simulink model "N3Z_tonetest14b"  (R2014b)
settings: Solver=ode3  SolverMode=SingleTasking  StartTime=0.0  StopTime=1e-4  FixedStep=fpgaclk  RelTol=1e-3
PreLoadFcn:
  | %fpgaclk=1/32.768e6
  | fpgaclk=1/49.162e6
  | 
  | SerialData=[1,zeros(1,11),1,0,0,1]
  | load ../N3workingG/window
  | win=win';  %Go back to using flatter and wider windowed sync function
  | %load ../N3workingG/hanning    %use Hahn window
  | 
  | load ../N3workingG/PREemphasis   %For pre-empasis and deemphasis FIRs
  | 
  | %LUT3=xls2LUT2('../IQI_Qdemod.xls'); LUT3
  | load ../N3workingG/LUT3
  | load ../N3workingG/FIRiq2
  | % xls2LUT
  | 
  | GetProgFiles
  | 
  | PinAssignments    %Get Pin references for TE0722
  | 
  | 
  | 
  | 
  | 
  | %LCD
  | LCDdata=[LCD_D7,LCD_D6,LCD_D5,LCD_D4,LCD_D3,LCD_D2,LCD_D1,LCD_D0] %Note MSB...LSB!
  | LCDctrl=[LCD_E,LCD_RW,LCD_RS];
  | 
  | %for RS232 on pins 3 and 5 of USBB
  | 
  | %BT chip connections for WT12
  | 
  | RX_BT=RXD
  | TX_BT=TXD
  | 
  | RST_BB=RES
  | 
  | %PCMC=PCMC
  | %PCMS=PCMS
  | %PCMI=PCMI
  | %PCMO=PCMO
  | 
  | %Aliases:
  | SRDBT=PCMI
  | STDBT=PCMO
  | SCLK_BT=PCMC
  | SFS_BT=PCMS
  | 
  | %ADC control
  | 
  | %SDOA=SDOA
  | %SDOB=SDOB
  | %SCK=SCK
  | CONV=Csbar
  | CAL=Cal
  | 
  | ADC_G=[ADC_G3,ADC_G2,ADC_G1,ADC_G0]
  | %PD settings hard coded now
  | 
  | %%%%%%
  | TX_LOW=TX_Low
  | ... (+11 lines)
StartFcn:
  | SerialData=[1,zeros(1,11),1,0,0,1]
values from neighbouring files (symbols this model uses):
  ADC_G0 = {'P10'}    [PinAssignments.m]
  ADC_G1 = {'P11'}    [PinAssignments.m]
  ADC_G2 = {'N14'}    [PinAssignments.m]
  ADC_G3 = {'M11'}    [PinAssignments.m]
  Cal = {'L12'}    [PinAssignments.m]
  Csbar = {'M12'}    [PinAssignments.m]
  LCD_D0 = {'J13'}    [PinAssignments.m]
  LCD_D1 = {'J14'}    [PinAssignments.m]
  LCD_D2 = {'F15'}    [PinAssignments.m]
  LCD_D3 = {'H14'}    [PinAssignments.m]
  LCD_D4 = {'G12'}    [PinAssignments.m]
  LCD_D5 = {'L15'}    [PinAssignments.m]
  LCD_D6 = {'M14'}    [PinAssignments.m]
  LCD_D7 = {'K15'}    [PinAssignments.m]
  PCMC = {'H11'}    [PinAssignments.m]
  PCMI = {'H12'}    [PinAssignments.m]
  PCMO = {'N13'}    [PinAssignments.m]
  PCMS = {'M10'}    [PinAssignments.m]
  RES = {'G11'}    [PinAssignments.m]
  RXD = {'H13'}    [PinAssignments.m]
  TX_Low = {'P15'}    [PinAssignments.m]
  TXD = {'P13'}    [PinAssignments.m]
undefined symbols (not defined in the file or in its folder): AXI4, FIRRX, FIRTX, Lite
libraries: xbsIndex_r4 x1214, MyFunctions x43
(part 5 of 9)

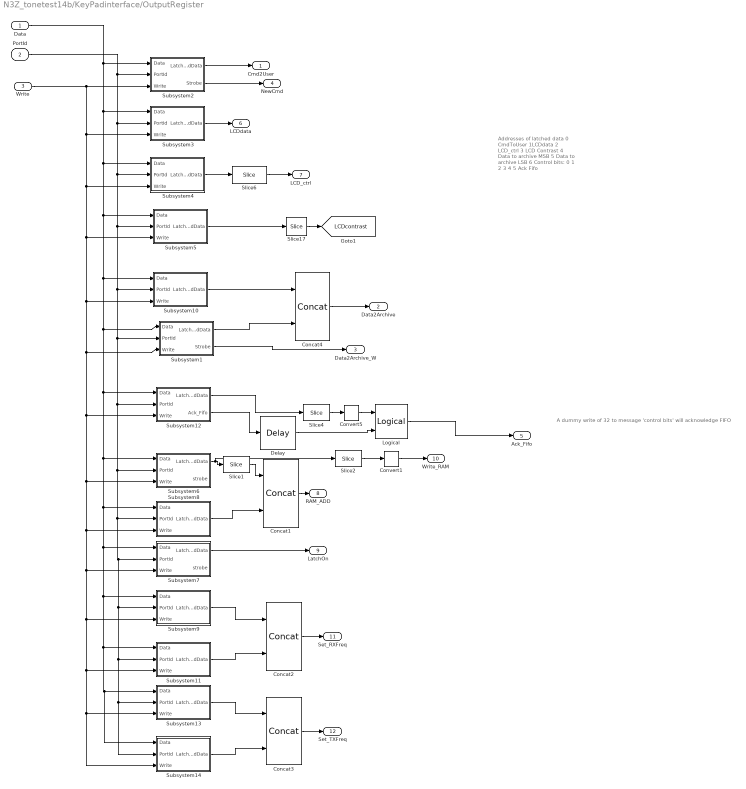
== system N3Z_tonetest14b/KeyPadinterface/OutputRegister ==
  note: A dummy write of 32 to message 'control bits' will acknowledge FIFO
  note: Addresses of latched data
      | 0 CmdToUser
      | 1LCDdata
      | 2 LCD_ctrl
      | 3 LCD Contrast
      | 4 Data to archive MSB
      | 5 Data to archive LSB
      | 6 Control bits:
      | 	0
      | 	1
      | 	2
      | 	3
      | 	4
      | 	5 Ack Fifo
  Data : Inport
  PortId : Inport  Port=2
  Write : Inport  Port=3
  Concat{1..4} (4 alike) : xbsIndex_r4/Concat  num_inputs=2  dbl_ovrd=off  block_type=concat
      settings: block_version=8.2.02
  Convert1 : xbsIndex_r4/Convert  gui_display_data_type=Fixed-point  arith_type=Boolean  n_bits=16  bin_pt=0  float_type=Single  exp_bits=8  fraction_bits=24  quantization=Truncate  overflow=Wrap  en=off  latency=0  pipeline=off  dbl_ovrd=off  block_type=convert
      settings: xl_area=[0, 0, 0, 0, 0, 0, 0]  block_version=VER_STRING_GOES_HERE
  Convert5 : xbsIndex_r4/Convert  gui_display_data_type=Fixed-point  arith_type=Boolean  n_bits=16  bin_pt=0  float_type=Single  exp_bits=8  fraction_bits=24  quantization=Truncate  overflow=Wrap  en=off  latency=0  pipeline=off  dbl_ovrd=off  block_type=convert
      settings: xl_area=[0, 0, 0, 0, 0, 0, 0]  block_version=VER_STRING_GOES_HERE
  Delay : xbsIndex_r4/Delay  rst=off  infoeditControl=Selection of Reset will increase slice count due to use of real FFs and instead of SRLs  en=off  latency=1  reg_retiming=off  dbl_ovrd=off  block_type=delay
      settings: infoedit=Hardware notes: A delay line is a chain, each link of which is an SRL16 followed by a flip-flop. If register retiming is enabled, the delay line is a chain of flip-flops.  block_version=8.2.02
  Logical : xbsIndex_r4/Logical  logical_function=AND  inputs=2  en=off  latency=0  precision=Full  arith_type=Unsigned  n_bits=16  bin_pt=0  align_bp=on  dbl_ovrd=off  block_type=logical
      settings: block_version=8.2.02
  Slice1 : xbsIndex_r4/Slice  nbits=2  boolean_output=off  mode=Lower Bit Location + Width  bit1=-16  base1=MSB of Input  bit0=0  base0=LSB of Input  dbl_ovrd=off  block_type=slice
      settings: block_version=VER_STRING_GOES_HERE
  Slice17 : xbsIndex_r4/Slice  nbits=6  boolean_output=off  mode=Lower Bit Location + Width  bit1=3  base1=MSB of Input  bit0=0  base0=LSB of Input  dbl_ovrd=off  block_type=slice
      settings: block_version=8.2.02
  Slice2 : xbsIndex_r4/Slice  nbits=1  boolean_output=off  mode=Lower Bit Location + Width  bit1=-16  base1=MSB of Input  bit0=2  base0=LSB of Input  dbl_ovrd=off  block_type=slice
      settings: block_version=VER_STRING_GOES_HERE
  Slice4 : xbsIndex_r4/Slice  nbits=1  boolean_output=off  mode=Lower Bit Location + Width  bit1=-16  base1=MSB of Input  bit0=5  base0=LSB of Input  dbl_ovrd=off  block_type=slice
      settings: block_version=VER_STRING_GOES_HERE
  Slice6 : xbsIndex_r4/Slice  nbits=4  boolean_output=off  mode=Lower Bit Location + Width  bit1=3  base1=MSB of Input  bit0=0  base0=LSB of Input  dbl_ovrd=off  block_type=slice
      settings: block_version=8.2.02
  Subsystem1 : Subsystem
  Subsystem10 : Subsystem
  Subsystem11 : Subsystem
  Subsystem12 : Subsystem
  Subsystem13 : Subsystem
  Subsystem14 : Subsystem
  Subsystem2 : Subsystem
  Subsystem3 : Subsystem
  Subsystem4 : Subsystem
  Subsystem5 : Subsystem
  Subsystem6 : Subsystem
  Subsystem7 : Subsystem
  Subsystem8 : Subsystem
  Subsystem9 : Subsystem
  Cmd2User : Outport
  Data2Archive : Outport  Port=2
  Data2Archive_W : Outport  Port=3
  NewCmd : Outport  Port=4
  Ack_Fifo : Outport  Port=5
  LCDdata : Outport  Port=6
  LCD_ctrl : Outport  Port=7
  RAM_ADD : Outport  Port=8
  LatchOn : Outport  Port=9
  Write_RAM : Outport  Port=10
  Set_RXFreq : Outport  Port=11
  Set_TXFreq : Outport  Port=12
  tag scope: LCDcontrast=global
  wires:
  PortId/1 -> Subsystem2/2(PortId), Subsystem3/2(PortId), Subsystem4/2(PortId), Subsystem5/2(PortId), Subsystem10/2(PortId), Subsystem1/2(PortId), Subsystem12/2(PortId), Subsystem8/2(PortId), Subsystem9/2(PortId), Subsystem11/2(PortId), Subsystem13/2(PortId), Subsystem14/2(PortId), Subsystem7/2(PortId), Subsystem6/2(PortId)
  Data/1 -> Subsystem2/1(Data), Subsystem3/1(Data), Subsystem4/1(Data), Subsystem5/1(Data), Subsystem10/1(Data), Subsystem1/1(Data), Subsystem12/1(Data), Subsystem8/1(Data), Subsystem14/1(Data), Subsystem13/1(Data), Subsystem11/1(Data), Subsystem9/1(Data), Subsystem7/1(Data), Subsystem6/1(Data)
  Write/1 -> Subsystem2/3(Write), Subsystem3/3(Write), Subsystem4/3(Write), Subsystem5/3(Write), Subsystem10/3(Write), Subsystem1/3(Write), Subsystem12/3(Write), Subsystem6/3(Write), Subsystem8/3(Write), Subsystem9/3(Write), Subsystem11/3(Write), Subsystem13/3(Write), Subsystem14/3(Write), Subsystem7/3(Write)
  Subsystem2/1(LatchedData) -> Cmd2User/1
  Concat4/1 -> Data2Archive/1
  Subsystem10/1(LatchedData) -> Concat4/1
  Subsystem12/1(LatchedData) -> Slice4/1
  Slice4/1 -> Convert5/1
  Convert5/1 -> Logical/1
  Subsystem2/2(Strobe) -> NewCmd/1
  Subsystem12/2(Ack_Fifo) -> Delay/1
  Logical/1 -> Ack_Fifo/1
  Delay/1 -> Logical/2
  Subsystem3/1(LatchedData) -> LCDdata/1
  Subsystem4/1(LatchedData) -> Slice6/1
  Slice6/1 -> LCD_ctrl/1
  Subsystem5/1(LatchedData) -> Slice17/1
  Slice17/1 -> [LCDcontrast]
  Subsystem1/2(Strobe) -> Data2Archive_W/1
  Subsystem1/1(LatchedData) -> Concat4/2
  Subsystem7/1(LatchedData) -> LatchOn/1
  Subsystem6/1(LatchedData) -> Slice1/1, Slice2/1
  Slice1/1 -> Concat1/1
  Subsystem8/1(LatchedData) -> Concat1/2
  Concat1/1 -> RAM_ADD/1
  Slice2/1 -> Convert1/1
  Convert1/1 -> Write_RAM/1
  Subsystem9/1(LatchedData) -> Concat2/1
  Subsystem11/1(LatchedData) -> Concat2/2
  Concat2/1 -> Set_RXFreq/1
  Subsystem13/1(LatchedData) -> Concat3/1
  Subsystem14/1(LatchedData) -> Concat3/2
  Concat3/1 -> Set_TXFreq/1

== system N3Z_tonetest14b/LoranPulsedetect/FastLevelMonitor ==
  note: Add 13 bits above and below to get ~2.5s time constant
  note: Feb 2011 added 1 bit to AddSub unit
  note: Increase Threshold 25%
  In1 : Inport
  En : Inport  Port=2
  AddSub : xbsIndex_r4/AddSub  mode=Addition or Subtraction  use_carryin=off  use_carryout=off  en=off  latency=0  precision=User Defined  arith_type=Unsigned  n_bits=13  bin_pt=0  quantization=Truncate  overflow=Wrap  use_behavioral_HDL=off  hw_selection=Fabric  pipelined=off  dbl_ovrd=off  block_type=addsub
      settings: block_version=12.2
  AddSub1 : xbsIndex_r4/AddSub  mode=Addition  use_carryin=off  use_carryout=off  en=off  latency=0  precision=User Defined  arith_type=Unsigned  n_bits=8  bin_pt=0  quantization=Truncate  overflow=Wrap  use_behavioral_HDL=off  hw_selection=Fabric  pipelined=off  dbl_ovrd=off  block_type=addsub
      settings: block_version=12.2
  Convert : xbsIndex_r4/Convert  gui_display_data_type=Fixed-point  arith_type=Boolean  n_bits=16  bin_pt=14  float_type=Single  exp_bits=8  fraction_bits=24  quantization=Truncate  overflow=Wrap  en=off  latency=0  pipeline=off  dbl_ovrd=off  block_type=convert
      settings: block_version=12.2
  Convert1 : xbsIndex_r4/Convert  gui_display_data_type=Fixed-point  arith_type=Boolean  n_bits=16  bin_pt=14  float_type=Single  exp_bits=8  fraction_bits=24  quantization=Truncate  overflow=Wrap  en=off  latency=0  pipeline=off  dbl_ovrd=off  block_type=convert
      settings: block_version=12.2
  Convert2 : xbsIndex_r4/Convert  gui_display_data_type=Fixed-point  arith_type="Signed  (2's comp)"  n_bits=8  bin_pt=0  float_type=Single  exp_bits=8  fraction_bits=24  quantization=Truncate  overflow=Wrap  en=off  latency=0  pipeline=off  dbl_ovrd=off  block_type=convert
      settings: block_version=12.2
  Counter : xbsIndex_r4/Counter  cnt_type=Free Running  cnt_to=Inf  operation=Up  start_count=0  cnt_by_val=1  arith_type=Unsigned  n_bits=8  bin_pt=0  load_pin=off  rst=off  en=on  explicit_period=on  period=fpgaclk  use_behavioral_HDL=off  implementation=Fabric  dbl_ovrd=off  block_type=counter
      settings: block_version=12.2
  Monostable : MyFunctions/Monostable
  Register : xbsIndex_r4/Register  init=0  rst=on  en=on  dbl_ovrd=off  block_type=register
      settings: block_version=12.2
  Register1 : xbsIndex_r4/Register  init=0  rst=off  en=on  dbl_ovrd=off  block_type=register
      settings: block_version=12.2
  Slice1 : xbsIndex_r4/Slice  nbits=1  boolean_output=off  mode=Upper Bit Location + Width  bit1=0  base1=MSB of Input  bit0=0  base0=LSB of Input  dbl_ovrd=off  block_type=slice
      settings: block_version=12.2
  Slice2 : xbsIndex_r4/Slice  nbits=1  boolean_output=off  mode=Upper Bit Location + Width  bit1=0  base1=MSB of Input  bit0=0  base0=LSB of Input  dbl_ovrd=off  block_type=slice
      settings: block_version=12.2
  Slice3 : xbsIndex_r4/Slice  nbits=8  boolean_output=off  mode=Upper Bit Location + Width  bit1=0  base1=MSB of Input  bit0=0  base0=LSB of Input  dbl_ovrd=off  block_type=slice
      settings: block_version=12.2
  Slice4 : xbsIndex_r4/Slice  nbits=8  boolean_output=off  mode=Upper Bit Location + Width  bit1=-1  base1=MSB of Input  bit0=0  base0=LSB of Input  dbl_ovrd=off  block_type=slice
      settings: block_version=12.2
  Slice5 : xbsIndex_r4/Slice  nbits=6  boolean_output=off  mode=Upper Bit Location + Width  bit1=0  base1=MSB of Input  bit0=0  base0=LSB of Input  dbl_ovrd=off  block_type=slice
      settings: block_version=12.2
  SignalLevel : Outport
  wires:
  In1/1 -> Slice1/1, Slice4/1
  AddSub/1 -> Register/1
  En/1 -> Register/3, Counter/1
  Slice1/1 -> Convert/1
  Convert/1 -> AddSub/3
  Register/1 -> AddSub/1, Slice3/1, Slice5/1
  Counter/1 -> Slice2/1
  Monostable/1 -> Convert1/1
  Convert1/1 -> Register/2, Register1/2
  Slice2/1 -> Monostable/1
  Register1/1 -> SignalLevel/1
  Slice4/1 -> Convert2/1
  Convert2/1 -> AddSub/2
  Slice3/1 -> AddSub1/1
  Slice5/1 -> AddSub1/2
  AddSub1/1 -> Register1/1

== system N3Z_tonetest14b/LoranPulsedetect/LoranTrigger ==
  note: Divides unsigned number by 2
  LoranSignal : Inport
  Thresh : Inport  Port=2
  Relational : xbsIndex_r4/Relational  mode=a>b  op_type=Bool  en=off  latency=1  dbl_ovrd=off  block_type=relational
      settings: block_version=12.2
  Slice : xbsIndex_r4/Slice  nbits=7  boolean_output=off  mode=Upper Bit Location + Width  bit1=0  base1=MSB of Input  bit0=0  base0=LSB of Input  dbl_ovrd=off  block_type=slice
      settings: block_version=12.2
  Trig : Outport
  wires:
  Slice/1 -> Relational/2
  LoranSignal/1 -> Relational/1
  Relational/1 -> Trig/1
  Thresh/1 -> Slice/1

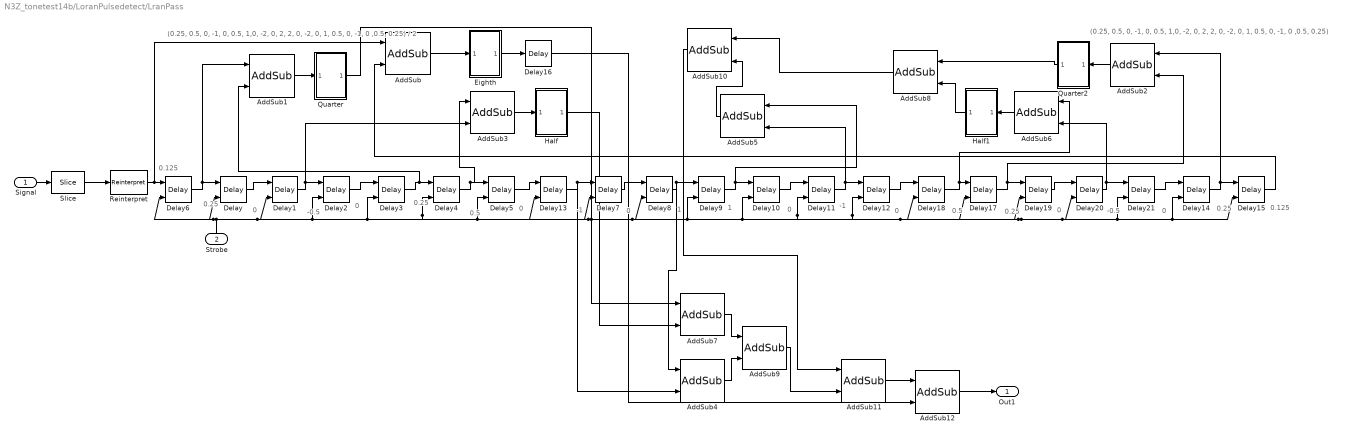
== system N3Z_tonetest14b/LoranPulsedetect/LranPass ==
  note: (0.25, 0.5, 0, -1, 0, 0.5, 1,0, -2, 0, 2, 2, 0, -2, 0, 1, 0.5, 0, -1, 0 ,0.5, 0.25) / 2
  note: (0.25, 0.5, 0, -1, 0, 0.5, 1,0, -2, 0, 2, 2, 0, -2, 0, 1, 0.5, 0, -1, 0 ,0.5, 0.25)
  note: 0.125
  note: 0.25
  note: 0
  note: -0.5
  note: 0
  note: 0.25
  note: 0.5
  note: 0
  note: -1
  note: 0
  note: 1
  note: 1
  note: 0
  note: -1
  note: 0
  note: 0.5
  note: 0.25
  note: 0
  note: -0.5
  note: 0
  note: 0.25
  note: 0.125
  Signal : Inport
  Strobe : Inport  Port=2
  AddSub{,1,7..10} (6 alike) : xbsIndex_r4/AddSub  mode=Addition  use_carryin=off  use_carryout=off  en=off  latency=1  precision=Full  arith_type=Unsigned  n_bits=16  bin_pt=14  quantization=Truncate  overflow=Wrap  use_behavioral_HDL=off  hw_selection=Fabric  pipelined=off  dbl_ovrd=off  block_type=addsub
      settings: block_version=12.2
  AddSub11 : xbsIndex_r4/AddSub  mode=Addition  use_carryin=off  use_carryout=off  en=off  latency=1  precision=User Defined  arith_type="Signed  (2's comp)"  n_bits=9  bin_pt=0  quantization=Truncate  overflow=Wrap  use_behavioral_HDL=off  hw_selection=Fabric  pipelined=off  dbl_ovrd=off  block_type=addsub
      settings: block_version=12.2
  AddSub12 : xbsIndex_r4/AddSub  mode=Addition  use_carryin=off  use_carryout=off  en=off  latency=1  precision=User Defined  arith_type="Signed  (2's comp)"  n_bits=9  bin_pt=0  quantization=Truncate  overflow=Wrap  use_behavioral_HDL=off  hw_selection=Fabric  pipelined=off  dbl_ovrd=off  block_type=addsub
      settings: block_version=12.2
  AddSub2 : xbsIndex_r4/AddSub  mode=Addition  use_carryin=off  use_carryout=off  en=off  latency=0  precision=Full  arith_type=Unsigned  n_bits=16  bin_pt=14  quantization=Truncate  overflow=Wrap  use_behavioral_HDL=off  hw_selection=Fabric  pipelined=off  dbl_ovrd=off  block_type=addsub
      settings: block_version=12.2
  AddSub{3..6} (4 alike) : xbsIndex_r4/AddSub  mode=Subtraction  use_carryin=off  use_carryout=off  en=off  latency=1  precision=Full  arith_type=Unsigned  n_bits=16  bin_pt=14  quantization=Truncate  overflow=Wrap  use_behavioral_HDL=off  hw_selection=Fabric  pipelined=off  dbl_ovrd=off  block_type=addsub
      settings: block_version=12.2
  Delay{,1..15,17..21} (21 alike) : xbsIndex_r4/Delay  rst=off  infoeditControl=Selection of Reset will increase slice count due to use of real FFs and instead of SRLs  en=on  latency=1  reg_retiming=off  dbl_ovrd=off  block_type=delay
      settings: block_version=12.2
  Delay16 : xbsIndex_r4/Delay  rst=off  infoeditControl=Selection of Reset will increase slice count due to use of real FFs and instead of SRLs  en=off  latency=3  reg_retiming=off  dbl_ovrd=off  block_type=delay
      settings: block_version=12.2
  Eighth : Subsystem
  Half : Subsystem
  Half1 : Subsystem
  Quarter : Subsystem
  Quarter2 : Subsystem
  Reinterpret : xbsIndex_r4/Reinterpret  force_arith_type=on  arith_type="Signed  (2's comp)"  force_bin_pt=off  bin_pt=0  block_type=reinterpret
      settings: infoedit="Changes signal type without altering the binary representation.   You can changed the signal between signed and unsigned, and relocate the binary point.<br><br>Hardware notes: In hardware this block costs nothing.<br><br>Example:  Suppose the input is 6 bits wide, signed, with 2 fractional bits, and the output is forced to unsigned with 0 fractional bits.  Then an input of -2.0 (1110.00 in binary 2's complement) becomes an output of 56 (111000 in binary)."  block_version=12.2
  Slice : xbsIndex_r4/Slice  nbits=8  boolean_output=off  mode=Upper Bit Location + Width  bit1=0  base1=MSB of Input  bit0=0  base0=LSB of Input  dbl_ovrd=off  block_type=slice
      settings: block_version=12.2
  Out1 : Outport
  wires:
  Delay6/1 -> Delay/1, AddSub1/1
  Delay/1 -> Delay1/1
  Delay1/1 -> Delay2/1, AddSub3/2
  Delay2/1 -> Delay3/1
  Delay3/1 -> Delay4/1, AddSub1/2
  Delay4/1 -> Delay5/1, AddSub3/1
  Strobe/1 -> Delay6/2, Delay/2, Delay1/2, Delay2/2, Delay3/2, Delay4/2, Delay5/2, Delay13/2, Delay7/2, Delay8/2, Delay9/2, Delay10/2, Delay11/2, Delay12/2, Delay18/2, Delay17/2, Delay19/2, Delay20/2, Delay21/2, Delay14/2, Delay15/2
  Signal/1 -> Slice/1
  Delay13/1 -> Delay7/1, AddSub4/2
  Delay7/1 -> Delay8/1
  Delay8/1 -> Delay9/1, AddSub4/1
  Delay9/1 -> Delay10/1, AddSub5/1
  Delay10/1 -> Delay11/1
  Delay11/1 -> Delay12/1, AddSub5/2
  Delay5/1 -> Delay13/1
  Slice/1 -> Reinterpret/1
  Delay17/1 -> Delay19/1, AddSub2/2
  Delay19/1 -> Delay20/1
  Delay20/1 -> Delay21/1, AddSub6/2
  Delay21/1 -> Delay14/1
  Delay14/1 -> Delay15/1, AddSub2/1
  Delay15/1 -> AddSub/2
  Delay18/1 -> Delay17/1, AddSub6/1
  Delay12/1 -> Delay18/1
  Reinterpret/1 -> Delay6/1, AddSub/1
  AddSub/1 -> Eighth/1(In1)
  AddSub2/1 -> Quarter2/1(In1)
  AddSub1/1 -> Quarter/1(In1)
  AddSub6/1 -> Half1/1(In1)
  AddSub3/1 -> Half/1(In1)
  Quarter/1(Out1) -> AddSub7/1
  Half/1(Out1) -> AddSub7/2
  Half1/1(Out1) -> AddSub8/2
  AddSub7/1 -> AddSub9/1
  AddSub4/1 -> AddSub9/2
  AddSub8/1 -> AddSub10/1
  AddSub5/1 -> AddSub10/2
  AddSub10/1 -> AddSub11/1
  AddSub9/1 -> AddSub11/2
  Eighth/1(Out1) -> Delay16/1
  AddSub11/1 -> AddSub12/1
  Delay16/1 -> AddSub12/2
  AddSub12/1 -> Out1/1
  Quarter2/1(Out1) -> AddSub8/1

== system N3Z_tonetest14b/SSBmodulator /RampGen ==
  note: Added 8 bits to get more precission on phase determination
  In1 : Inport
  Accumulator : xbsIndex_r4/Accumulator  operation=Add  n_bits=21  overflow=Wrap  scale=1  rst=off  hasbypass=off  infoeditControl=reset for floating point data type must be asserted for a minimum of 2 cycles  en=off  latency=0  msb_inp=100  msb=100  lsb=-100  use_behavioral_HDL=on  implementation=Fabric  dbl_ovrd=off  block_type=accum
      settings: block_version=VER_STRING_GOES_HERE
  Slice : xbsIndex_r4/Slice  nbits=17  boolean_output=off  mode=Upper Bit Location + Width  bit1=0  base1=MSB of Input  bit0=0  base0=LSB of Input  dbl_ovrd=off  block_type=slice
      settings: block_version=VER_STRING_GOES_HERE
  Out1 : Outport
  wires:
  Accumulator/1 -> Slice/1
  In1/1 -> Accumulator/1
  Slice/1 -> Out1/1

== system N3Z_tonetest14b/SSBmodulator /Subsystem ==
  note: Ramp from -2^15 to +2^15
  In1 : Inport
  In3 : Inport  Port=2
  AddSub : xbsIndex_r4/AddSub  mode=Subtraction  use_carryin=off  use_carryout=off  en=off  latency=0  precision=Full  arith_type=Unsigned  n_bits=16  bin_pt=14  quantization=Truncate  overflow=Wrap  use_behavioral_HDL=off  hw_selection=Fabric  pipelined=off  use_rpm=on  dbl_ovrd=off  block_type=addsub
      settings: block_version=VER_STRING_GOES_HERE
  Concat : xbsIndex_r4/Concat  num_inputs=2  dbl_ovrd=off  block_type=concat
      settings: block_version=VER_STRING_GOES_HERE
  Constant : xbsIndex_r4/Constant  const=0  gui_display_data_type=Fixed-point  arith_type=Signed (2's comp)  n_bits=8  bin_pt=0  preci_type=Single  exp_width=8  frac_width=24  explicit_period=on  period=fpgaclk  equ=P=C  opselect=C  inp2=PCIN>>17  opr=+  inp1=P  carry=CIN  dbl_ovrd=off  block_type=constant
      settings: block_version=VER_STRING_GOES_HERE
  Inverter : xbsIndex_r4/Inverter  en=off  latency=0  dbl_ovrd=off  block_type=inv
      settings: block_version=VER_STRING_GOES_HERE
  Logical : xbsIndex_r4/Logical  logical_function=AND  inputs=2  en=off  latency=1  precision=Full  arith_type=Unsigned  n_bits=16  bin_pt=0  align_bp=on  dbl_ovrd=off  block_type=logical
      settings: block_version=VER_STRING_GOES_HERE
  Reinterpret : xbsIndex_r4/Reinterpret  force_arith_type=on  arith_type="Signed  (2's comp)"  force_bin_pt=on  bin_pt=0  block_type=cast
      settings: infoedit="Changes signal type without altering the binary representation.   You can changed the signal between signed and unsigned, and relocate the binary point.<br><br>Hardware notes: In hardware this block costs nothing.<br><br>Example:  Suppose the input is 6 bits wide, signed, with 2 fractional bits, and the output is forced to unsigned with 0 fractional bits.  Then an input of -2.0 (1110.00 in binary 2's complement) becomes an output of 56 (111000 in binary)."  block_version=VER_STRING_GOES_HERE
  Relational : xbsIndex_r4/Relational  mode=a>b  op_type=Bool  en=off  latency=1  dbl_ovrd=off  block_type=relational
      settings: block_version=VER_STRING_GOES_HERE
  Relational1 : xbsIndex_r4/Relational  mode=a>b  op_type=Bool  en=off  latency=1  dbl_ovrd=off  block_type=relational
      settings: block_version=VER_STRING_GOES_HERE
  Slice : xbsIndex_r4/Slice  nbits=15  boolean_output=off  mode=Upper Bit Location + Width  bit1=-2  base1=MSB of Input  bit0=0  base0=LSB of Input  dbl_ovrd=off  block_type=slice
      settings: block_version=VER_STRING_GOES_HERE
  Slice1 : xbsIndex_r4/Slice  nbits=1  boolean_output=off  mode=Upper Bit Location + Width  bit1=-1  base1=MSB of Input  bit0=0  base0=LSB of Input  dbl_ovrd=off  block_type=slice
      settings: block_version=VER_STRING_GOES_HERE
  Slice2 : xbsIndex_r4/Slice  nbits=1  boolean_output=off  mode=Upper Bit Location + Width  bit1=0  base1=MSB of Input  bit0=0  base0=LSB of Input  dbl_ovrd=off  block_type=slice
      settings: block_version=VER_STRING_GOES_HERE
  Out1 : Outport
  Polarity : Outport  Port=2
  wires:
  Constant/1 -> AddSub/1
  AddSub/1 -> Relational1/2
  Relational/1 -> Logical/1
  Relational1/1 -> Logical/2
  In1/1 -> AddSub/2, Relational/1
  Logical/1 -> Out1/1
  In3/1 -> Slice/1, Slice2/1, Slice1/1
  Slice/1 -> Concat/2
  Slice1/1 -> Inverter/1
  Inverter/1 -> Concat/1
  Concat/1 -> Reinterpret/1
  Reinterpret/1 -> Relational/2, Relational1/1
  Slice2/1 -> Polarity/1

== system N3Z_tonetest14b/Subsystem1/Subsystem1 ==
  note: April 09, increased delay to latch ADC value to get another bit?
  SDOA : Inport
  SCK : Inport  Port=2
  Conv : Inport  Port=3
  Concat : xbsIndex_r4/Concat  num_inputs=2  dbl_ovrd=off  block_type=concat
      settings: block_version=VER_STRING_GOES_HERE
  Inverter : xbsIndex_r4/Inverter  en=off  latency=0  dbl_ovrd=off  block_type=inv
      settings: block_version=9.2.01
  Monostable1 : MyFunctions/Monostable
  Monostable2 : MyFunctions/Monostable
  Register : xbsIndex_r4/Register  init=0  rst=on  en=on  dbl_ovrd=off  block_type=register
      settings: xl_area=[8 16 0 0 0 0 0]  block_version=VER_STRING_GOES_HERE
  Register1 : xbsIndex_r4/Register  init=0  rst=off  en=on  dbl_ovrd=off  block_type=register
      settings: xl_area=[8 16 0 0 0 0 0]  block_version=VER_STRING_GOES_HERE
  Reinterpret : xbsIndex_r4/Reinterpret  force_arith_type=on  arith_type="Signed  (2's comp)"  force_bin_pt=off  bin_pt=0  block_type=reinterpret
      settings: infoedit="Changes signal type without altering the binary representation.   You can changed the signal between signed and unsigned, and relocate the binary point.<br><br>Hardware notes: In hardware this block costs nothing.<br><br>Example:  Suppose the input is 6 bits wide, signed, with 2 fractional bits, and the output is forced to unsigned with 0 fractional bits.  Then an input of -2.0 (1110.00 in binary 2's complement) becomes an output of 56 (111000 in binary)."  block_version=9.2.01
  Slice : xbsIndex_r4/Slice  nbits=15  boolean_output=off  mode=Lower Bit Location + Width  bit1=0  base1=MSB of Input  bit0=0  base0=LSB of Input  dbl_ovrd=off  block_type=slice
      settings: block_version=VER_STRING_GOES_HERE
  ADCValueA : Outport
  wires:
  Register/1 -> Slice/1
  Concat/1 -> Register/1, Register1/1
  Register1/1 -> Reinterpret/1
  SCK/1 -> Inverter/1
  Conv/1 -> Monostable1/1
  Monostable1/1 -> Register/2, Register1/2
  Monostable2/1 -> Register/3
  Inverter/1 -> Monostable2/1
  SDOA/1 -> Concat/2
  Reinterpret/1 -> ADCValueA/1
  Slice/1 -> Concat/1

== system N3Z_tonetest14b/Subsystem2/Divide2 ==
  note: Divide signed number by 2
  In1 : Inport
  Concat1 : xbsIndex_r4/Concat  num_inputs=2  dbl_ovrd=off  block_type=concat
      settings: block_version=12.2
  Reinterpret : xbsIndex_r4/Reinterpret  force_arith_type=on  arith_type="Signed  (2's comp)"  force_bin_pt=on  bin_pt=15  block_type=reinterpret
      settings: infoedit="Changes signal type without altering the binary representation.   You can changed the signal between signed and unsigned, and relocate the binary point.<br><br>Hardware notes: In hardware this block costs nothing.<br><br>Example:  Suppose the input is 6 bits wide, signed, with 2 fractional bits, and the output is forced to unsigned with 0 fractional bits.  Then an input of -2.0 (1110.00 in binary 2's complement) becomes an output of 56 (111000 in binary)."  block_version=8.2.02
  Slice1 : xbsIndex_r4/Slice  nbits=15  boolean_output=off  mode=Upper Bit Location + Width  bit1=0  base1=MSB of Input  bit0=0  base0=LSB of Input  dbl_ovrd=off  block_type=slice
      settings: block_version=12.2
  Slice4 : xbsIndex_r4/Slice  nbits=1  boolean_output=off  mode=Upper Bit Location + Width  bit1=0  base1=MSB of Input  bit0=0  base0=LSB of Input  dbl_ovrd=off  block_type=slice
      settings: block_version=12.2
  Out1 : Outport
  wires:
  Slice4/1 -> Concat1/1
  Slice1/1 -> Concat1/2
  Concat1/1 -> Reinterpret/1
  In1/1 -> Slice4/1, Slice1/1
  Reinterpret/1 -> Out1/1

== system N3Z_tonetest14b/Subsystem4/PCMclock ==
  note: 214748 to generate 512kHz with 40MHz clock
      | or 53687 for 128kHz
      | but 67109 for 32MHz clock!
      | 43691 for 49.152MHz
  Constant : xbsIndex_r4/Constant  const=4  gui_display_data_type=Fixed-point  arith_type=Unsigned  n_bits=4  bin_pt=0  preci_type=Single  exp_width=8  frac_width=24  explicit_period=on  period=fpgaclk  equ=P=C  opselect=C  inp2=PCIN>>17  opr=+  inp1=P  carry=CIN  dbl_ovrd=off  block_type=constant
      settings: block_version=9.2.01
  Constant2 : xbsIndex_r4/Constant  const=15  gui_display_data_type=Fixed-point  arith_type=Unsigned  n_bits=4  bin_pt=0  preci_type=Single  exp_width=8  frac_width=24  explicit_period=on  period=fpgaclk  equ=P=C  opselect=C  inp2=PCIN>>17  opr=+  inp1=P  carry=CIN  dbl_ovrd=off  block_type=constant
      settings: block_version=9.2.01
  Convert1 : xbsIndex_r4/Convert  gui_display_data_type=Fixed-point  arith_type=Boolean  n_bits=16  bin_pt=14  float_type=Single  exp_bits=8  fraction_bits=24  quantization=Truncate  overflow=Wrap  en=off  latency=0  pipeline=off  dbl_ovrd=off  block_type=convert
      settings: block_version=9.2.01
  Counter : xbsIndex_r4/Counter  cnt_type=Free Running  cnt_to=Inf  operation=Up  start_count=0  cnt_by_val=1  arith_type=Unsigned  n_bits=4  bin_pt=0  load_pin=off  rst=off  en=on  explicit_period=on  period=fpgaclk  use_behavioral_HDL=off  implementation=Fabric  use_rpm=off  dbl_ovrd=off  block_type=counter
      settings: block_version=9.2.01
  Delay : xbsIndex_r4/Delay  rst=off  infoeditControl=Selection of Reset will increase slice count due to use of real FFs and instead of SRLs  en=off  latency=2  reg_retiming=off  dbl_ovrd=off  block_type=delay
      settings: block_version=9.2.01
  Monostable1 : MyFunctions/Monostable
  Relational : xbsIndex_r4/Relational  mode=a<b  op_type=Bool  en=off  latency=1  dbl_ovrd=off  block_type=relational
      settings: block_version=9.2.01
  Relational1 : xbsIndex_r4/Relational  mode=a=b  op_type=Bool  en=off  latency=1  dbl_ovrd=off  block_type=relational
      settings: block_version=9.2.01
  128kHz : Outport
  Clk8kHz : Outport  Port=2
  STFS : Outport  Port=3
  wires:
  [Square128kHz] -> Monostable1/1, Delay/1
  Relational/1 -> Clk8kHz/1
  Constant/1 -> Relational/2
  Monostable1/1 -> Convert1/1
  Counter/1 -> Relational/1, Relational1/1
  Convert1/1 -> Counter/1
  Delay/1 -> 128kHz/1
  Constant2/1 -> Relational1/2
  Relational1/1 -> STFS/1

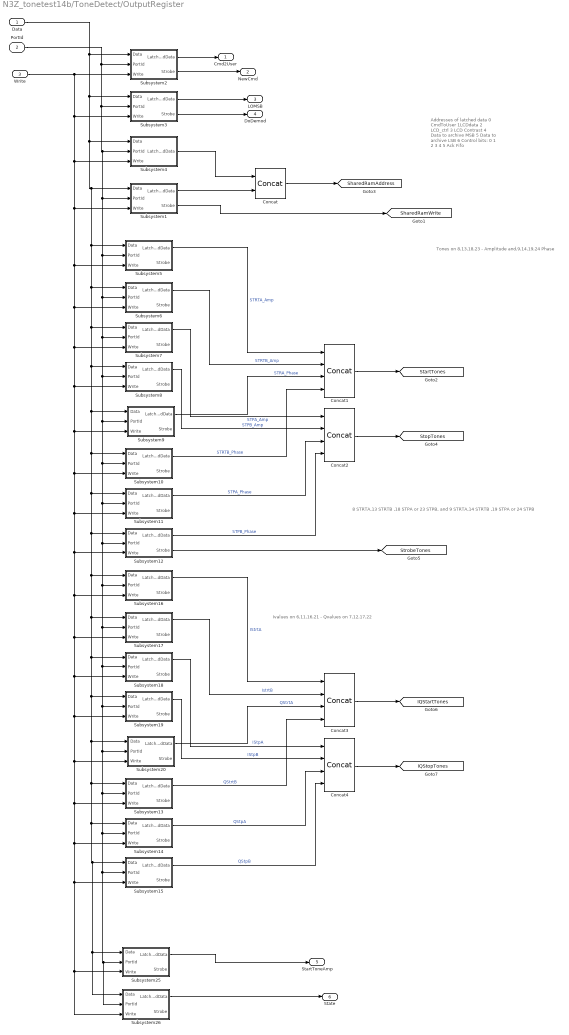
== system N3Z_tonetest14b/ToneDetect/OutputRegister ==
  note: 8 STRTA,13 STRTB ,18 STPA or 23 STPB, and 9 STRTA,14 STRTB ,19 STPA or 24 STPB
  note: Tones on 8,13,18,23 - Amplitude and,9,14,19,24 Phase
  note: Addresses of latched data
      | 0 CmdToUser
      | 1LCDdata
      | 2 LCD_ctrl
      | 3 LCD Contrast
      | 4 Data to archive MSB
      | 5 Data to archive LSB
      | 6 Control bits:
      | 	0
      | 	1
      | 	2
      | 	3
      | 	4
      | 	5 Ack Fifo
  note: Ivalues on 6,11,16,21 - Qvalues on 7,12,17,22
  Data : Inport
  PortId : Inport  Port=2
  Write : Inport  Port=3
  Concat : xbsIndex_r4/Concat  num_inputs=2  dbl_ovrd=off  block_type=concat
  Concat{1..4} (4 alike) : xbsIndex_r4/Concat  num_inputs=4  dbl_ovrd=off  block_type=concat
  Subsystem1 : Subsystem
  Subsystem10 : Subsystem
  Subsystem11 : Subsystem
  Subsystem12 : Subsystem
  Subsystem13 : Subsystem
  Subsystem14 : Subsystem
  Subsystem15 : Subsystem
  Subsystem16 : Subsystem
  Subsystem17 : Subsystem
  Subsystem18 : Subsystem
  Subsystem19 : Subsystem
  Subsystem2 : Subsystem
  Subsystem20 : Subsystem
  Subsystem25 : Subsystem
  Subsystem26 : Subsystem
  Subsystem3 : Subsystem
  Subsystem4 : Subsystem
  Subsystem5 : Subsystem
  Subsystem6 : Subsystem
  Subsystem7 : Subsystem
  Subsystem8 : Subsystem
  Subsystem9 : Subsystem
  Cmd2User : Outport
  NewCmd : Outport  Port=2
  LOMSB : Outport  Port=3
  DoDemod : Outport  Port=4
  StartToneAmp : Outport  Port=5
  State : Outport  Port=6
  tag scope: IQStartTones=global, IQStopTones=global, SharedRamAddress=global, SharedRamWrite=global, StartTones=global, StopTones=global, StrobeTones=global
  wires:
  Subsystem2/1(LatchedData) -> Cmd2User/1
  Subsystem2/2(Strobe) -> NewCmd/1
  Subsystem3/1(LatchedData) -> LOMSB/1
  Subsystem3/2(Strobe) -> DoDemod/1
  Subsystem4/1(LatchedData) -> Concat/1
  Subsystem1/1(LatchedData) -> Concat/2
  Subsystem1/2(Strobe) -> [SharedRamWrite]
  Concat/1 -> [SharedRamAddress]
  Subsystem5/1(LatchedData) -> Concat1/1  "STRTA_Amp"
  Subsystem6/1(LatchedData) -> Concat1/2  "STRTB_Amp"
  Subsystem9/1(LatchedData) -> Concat1/3  "STRA_Phase"
  Subsystem10/1(LatchedData) -> Concat1/4  "STRTB_Phase"
  Concat1/1 -> [StartTones]
  Concat2/1 -> [StopTones]
  Subsystem7/1(LatchedData) -> Concat2/1  "STPA_Amp"
  Subsystem8/1(LatchedData) -> Concat2/2  "STPB_Amp"
  Subsystem11/1(LatchedData) -> Concat2/3  "STPA_Phase"
  Subsystem12/1(LatchedData) -> Concat2/4  "STPB_Phase"
  Subsystem12/2(Strobe) -> [StrobeTones]
  PortId/1 -> Subsystem2/2(PortId), Subsystem3/2(PortId), Subsystem5/2(PortId), Subsystem6/2(PortId), Subsystem7/2(PortId), Subsystem8/2(PortId), Subsystem9/2(PortId), Subsystem10/2(PortId), Subsystem11/2(PortId), Subsystem26/2(PortId), Subsystem25/2(PortId), Subsystem15/2(PortId), Subsystem14/2(PortId), Subsystem13/2(PortId), Subsystem20/2(PortId), Subsystem19/2(PortId), Subsystem18/2(PortId), Subsystem17/2(PortId), Subsystem16/2(PortId), Subsystem12/2(PortId), Subsystem1/2(PortId), Subsystem4/2(PortId)
  Data/1 -> Subsystem2/1(Data), Subsystem3/1(Data), Subsystem8/1(Data), Subsystem9/1(Data), Subsystem10/1(Data), Subsystem11/1(Data), Subsystem14/1(Data), Subsystem26/1(Data), Subsystem25/1(Data), Subsystem15/1(Data), Subsystem13/1(Data), Subsystem20/1(Data), Subsystem19/1(Data), Subsystem18/1(Data), Subsystem17/1(Data), Subsystem16/1(Data), Subsystem12/1(Data), Subsystem7/1(Data), Subsystem6/1(Data), Subsystem5/1(Data), Subsystem1/1(Data), Subsystem4/1(Data)
  Write/1 -> Subsystem2/3(Write), Subsystem3/3(Write), Subsystem5/3(Write), Subsystem6/3(Write), Subsystem7/3(Write), Subsystem8/3(Write), Subsystem9/3(Write), Subsystem10/3(Write), Subsystem11/3(Write), Subsystem15/3(Write), Subsystem25/3(Write), Subsystem26/3(Write), Subsystem14/3(Write), Subsystem13/3(Write), Subsystem20/3(Write), Subsystem19/3(Write), Subsystem18/3(Write), Subsystem17/3(Write), Subsystem16/3(Write), Subsystem12/3(Write), Subsystem1/3(Write), Subsystem4/3(Write)
  Subsystem16/1(LatchedData) -> Concat3/1  "IStrtA"
  Subsystem17/1(LatchedData) -> Concat3/2  "IstrtB"
  Subsystem20/1(LatchedData) -> Concat3/3  "QStrtA"
  Subsystem13/1(LatchedData) -> Concat3/4  "QStrtB"
  Concat3/1 -> [IQStartTones]
  Concat4/1 -> [IQStopTones]
  Subsystem18/1(LatchedData) -> Concat4/1  "IStpA"
  Subsystem19/1(LatchedData) -> Concat4/2  "IStpB"
  Subsystem14/1(LatchedData) -> Concat4/3  "QStpA"
  Subsystem15/1(LatchedData) -> Concat4/4  "QStpB"
  Subsystem25/1(LatchedData) -> StartToneAmp/1
  Subsystem26/1(LatchedData) -> State/1

== system N3Z_tonetest14b/User_Interface/Buffer ==
  note: When code is < 128, then code is valid ie buffer not empty.
  note: To acknowledge - need to do a dummy write!
  Cmd : Inport
  NewCmd : Inport  Port=2
  AckFifo : Inport  Port=3
  Concat : xbsIndex_r4/Concat  num_inputs=2  dbl_ovrd=off  block_type=concat
      settings: block_version=8.2.02
  Convert2 : xbsIndex_r4/Convert  gui_display_data_type=Fixed-point  arith_type=Boolean  n_bits=16  bin_pt=0  float_type=Single  exp_bits=8  fraction_bits=24  quantization=Truncate  overflow=Wrap  en=off  latency=0  pipeline=off  dbl_ovrd=off  block_type=convert
      settings: xl_area=[0, 0, 0, 0, 0, 0, 0]  block_version=VER_STRING_GOES_HERE
  Delay : xbsIndex_r4/Delay  rst=off  infoeditControl=Selection of Reset will increase slice count due to use of real FFs and instead of SRLs  en=off  latency=2  reg_retiming=off  dbl_ovrd=off  block_type=delay
      settings: infoedit=Hardware notes: A delay line is a chain, each link of which is an SRL16 followed by a flip-flop. If register retiming is enabled, the delay line is a chain of flip-flops.  block_version=8.2.02
  FIFO : xbsIndex_r4/FIFO  mem_type=Distributed RAM  performance_options=Standard_FIFO  embedded_registers=off  depth=16  percent_nbits=1  rst=off  rst_latency=1  en=off  use_dcount=off  use_percent_full_port=on  use_almost_empty=off  almost_empty_thresh=2  use_almost_full=off  almost_full_thresh=14  explicit_period=off  dbl_ovrd=off  block_type=fifo
      settings: block_version=8.2.02
  Slice : xbsIndex_r4/Slice  nbits=7  boolean_output=off  mode=Lower Bit Location + Width  bit1=0  base1=MSB of Input  bit0=0  base0=LSB of Input  dbl_ovrd=off  block_type=slice
      settings: infoedit="Extracts a given range of bits from each input sample and presents it at the output.  The output type is ordinarily unsigned with binary point at zero, but can be Boolean when the slice is one bit wide.<P><P>Hardware notes: In hardware this block costs nothing."  block_version=8.2.02
  CmdOut : Outport
  tag scope: DSP2UserFIFOfull=global
  wires:
  Cmd/1 -> FIFO/1
  NewCmd/1 -> Delay/1
  Slice/1 -> Concat/2
  FIFO/1 -> Slice/1
  Concat/1 -> CmdOut/1
  FIFO/2 -> Concat/1
  Delay/1 -> FIFO/2
  AckFifo/1 -> Convert2/1
  Convert2/1 -> FIFO/3
  FIFO/4 -> [DSP2UserFIFOfull]

== system N3Z_tonetest14b/User_Interface/Buffer2 ==
  note: When code is < 128, then code is valid ie buffer not empty.
  note: To acknowledge - need to do a dummy write!
  Cmd : Inport
  NewCmd : Inport  Port=2
  AckFifo : Inport  Port=3
  Concat : xbsIndex_r4/Concat  num_inputs=2  dbl_ovrd=off  block_type=concat
      settings: block_version=8.2.02
  Convert2 : xbsIndex_r4/Convert  gui_display_data_type=Fixed-point  arith_type=Boolean  n_bits=16  bin_pt=0  float_type=Single  exp_bits=8  fraction_bits=24  quantization=Truncate  overflow=Wrap  en=off  latency=0  pipeline=off  dbl_ovrd=off  block_type=convert
      settings: xl_area=[0, 0, 0, 0, 0, 0, 0]  block_version=VER_STRING_GOES_HERE
  Delay : xbsIndex_r4/Delay  rst=off  infoeditControl=Selection of Reset will increase slice count due to use of real FFs and instead of SRLs  en=off  latency=2  reg_retiming=off  dbl_ovrd=off  block_type=delay
      settings: infoedit=Hardware notes: A delay line is a chain, each link of which is an SRL16 followed by a flip-flop. If register retiming is enabled, the delay line is a chain of flip-flops.  block_version=8.2.02
  FIFO : xbsIndex_r4/FIFO  mem_type=Distributed RAM  performance_options=Standard_FIFO  embedded_registers=off  depth=16  percent_nbits=1  rst=off  rst_latency=1  en=off  use_dcount=off  use_percent_full_port=on  use_almost_empty=off  almost_empty_thresh=2  use_almost_full=off  almost_full_thresh=14  explicit_period=off  dbl_ovrd=off  block_type=fifo
      settings: block_version=8.2.02
  Slice : xbsIndex_r4/Slice  nbits=7  boolean_output=off  mode=Lower Bit Location + Width  bit1=0  base1=MSB of Input  bit0=0  base0=LSB of Input  dbl_ovrd=off  block_type=slice
      settings: infoedit="Extracts a given range of bits from each input sample and presents it at the output.  The output type is ordinarily unsigned with binary point at zero, but can be Boolean when the slice is one bit wide.<P><P>Hardware notes: In hardware this block costs nothing."  block_version=8.2.02
  CmdOut : Outport
  tag scope: KP2UserFIFOfull=global
  wires:
  Cmd/1 -> FIFO/1
  NewCmd/1 -> Delay/1
  Slice/1 -> Concat/2
  FIFO/1 -> Slice/1
  Concat/1 -> CmdOut/1
  FIFO/2 -> Concat/1
  Delay/1 -> FIFO/2
  AckFifo/1 -> Convert2/1
  Convert2/1 -> FIFO/3
  FIFO/4 -> [KP2UserFIFOfull]

== system N3Z_tonetest14b/User_Interface/Buffer3 ==
  note: When code is < 128, then code is valid ie buffer not empty.
  note: To acknowledge - need to do a dummy write!
  Cmd : Inport
  NewCmd : Inport  Port=2
  AckFifo : Inport  Port=3
  Concat : xbsIndex_r4/Concat  num_inputs=2  dbl_ovrd=off  block_type=concat
      settings: block_version=8.2.02
  Convert2 : xbsIndex_r4/Convert  gui_display_data_type=Fixed-point  arith_type=Boolean  n_bits=16  bin_pt=0  float_type=Single  exp_bits=8  fraction_bits=24  quantization=Truncate  overflow=Wrap  en=off  latency=0  pipeline=off  dbl_ovrd=off  block_type=convert
      settings: xl_area=[0, 0, 0, 0, 0, 0, 0]  block_version=VER_STRING_GOES_HERE
  Delay : xbsIndex_r4/Delay  rst=off  infoeditControl=Selection of Reset will increase slice count due to use of real FFs and instead of SRLs  en=off  latency=2  reg_retiming=off  dbl_ovrd=off  block_type=delay
      settings: infoedit=Hardware notes: A delay line is a chain, each link of which is an SRL16 followed by a flip-flop. If register retiming is enabled, the delay line is a chain of flip-flops.  block_version=8.2.02
  FIFO : xbsIndex_r4/FIFO  mem_type=Distributed RAM  performance_options=Standard_FIFO  embedded_registers=off  depth=16  percent_nbits=1  rst=off  rst_latency=1  en=off  use_dcount=off  use_percent_full_port=on  use_almost_empty=off  almost_empty_thresh=2  use_almost_full=off  almost_full_thresh=14  explicit_period=off  dbl_ovrd=off  block_type=fifo
      settings: block_version=8.2.02
  Slice : xbsIndex_r4/Slice  nbits=7  boolean_output=off  mode=Lower Bit Location + Width  bit1=0  base1=MSB of Input  bit0=0  base0=LSB of Input  dbl_ovrd=off  block_type=slice
      settings: infoedit="Extracts a given range of bits from each input sample and presents it at the output.  The output type is ordinarily unsigned with binary point at zero, but can be Boolean when the slice is one bit wide.<P><P>Hardware notes: In hardware this block costs nothing."  block_version=8.2.02
  CmdOut : Outport
  tag scope: TD2UserFIFOfull=global
  wires:
  Cmd/1 -> FIFO/1
  NewCmd/1 -> Delay/1
  Slice/1 -> Concat/2
  FIFO/1 -> Slice/1
  Concat/1 -> CmdOut/1
  FIFO/2 -> Concat/1
  Delay/1 -> FIFO/2
  AckFifo/1 -> Convert2/1
  Convert2/1 -> FIFO/3
  FIFO/4 -> [TD2UserFIFOfull]
